simulink model "iabcde_id1q1"  (R2017b)
settings: Solver=VariableStepAuto  StartTime=0.0  StopTime=10.0  RelTol=1e-3
settings Model: Creator=Lei  LastModifiedBy=Lei

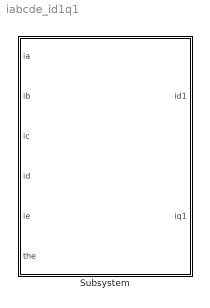
== system iabcde_id1q1 ==
  Subsystem : Subsystem

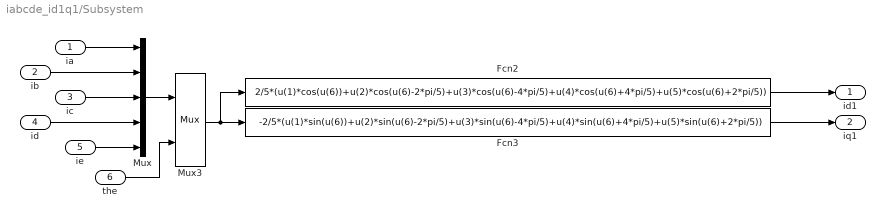
== system iabcde_id1q1/Subsystem ==
  ia : Inport
  ib : Inport  Port=2
  ic : Inport  Port=3
  id : Inport  Port=4
  ie : Inport  Port=5
  the : Inport  Port=6
  Fcn2 : Fcn  Expr=2/5*(u(1)*cos(u(6))+u(2)*cos(u(6)-2*pi/5)+u(3)*cos(u(6)-4*pi/5)+u(4)*cos(u(6)+4*pi/5)+u(5)*cos(u(6)+2*pi/5))
  Fcn3 : Fcn  Expr=-2/5*(u(1)*sin(u(6))+u(2)*sin(u(6)-2*pi/5)+u(3)*sin(u(6)-4*pi/5)+u(4)*sin(u(6)+4*pi/5)+u(5)*sin(u(6)+2*pi/5))
  Mux : Mux  Inputs=5
  Mux3 : Mux  Inputs=[5 1]
  id1 : Outport  InitialOutput=0
  iq1 : Outport  Port=2  InitialOutput=0
  wires:
  id/1 -> Mux/4
  ia/1 -> Mux/1
  ic/1 -> Mux/3
  ib/1 -> Mux/2
  ie/1 -> Mux/5
  the/1 -> Mux3/2
  Mux/1 -> Mux3/1
  Fcn2/1 -> id1/1
  Mux3/1 -> Fcn3/1, Fcn2/1
  Fcn3/1 -> iq1/1
